simulink subsystem "Channel_FIFO"  (R2024a)
settings: Solver=VariableStepAuto  StartTime=0.0  StopTime=10.0  RelTol=1e-3
model mask{Index=0}
libraries: hdlsllib x2, simulink x1
settings Model: Creator=versal  LastModifiedBy=versal

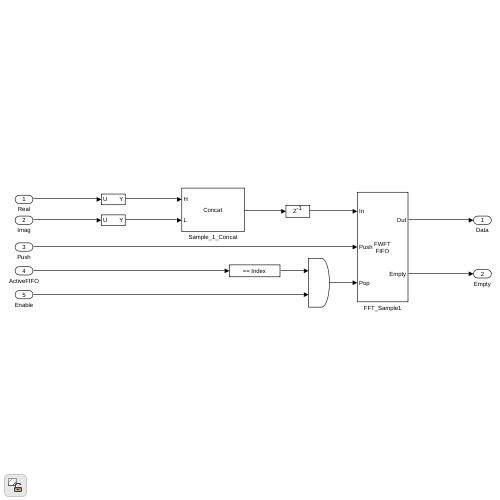
[thumbnail: Simulink's stored preview of the top-level diagram]
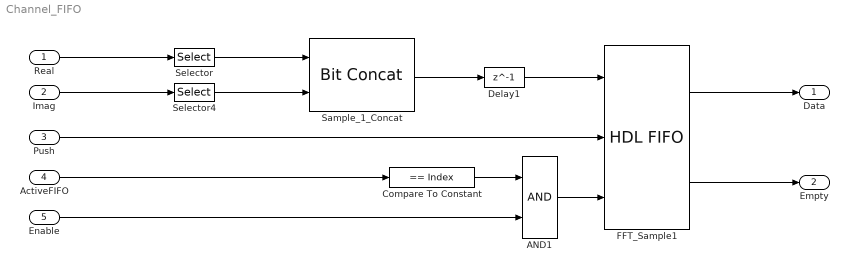
== system Channel_FIFO ==
  Real : Inport
  Imag : Inport  Port=2
  Push : Inport  Port=3
  ActiveFIFO : Inport  Port=4
  Enable : Inport  Port=5
  AND1 : Logic  IconShape=distinctive  AllPortsSameDT=off  OutDataTypeStr=boolean
  Compare To Constant : simulink/Logic and Bit Operations/Compare To Constant  relop===  const=Index  OutDataTypeStr=boolean
  Delay1 : Delay  DelayLength=1
  FFT_Sample1 : hdlsllib/HDL RAMs/HDL FIFO  fifo_size=128  mode=FWFT  ratio=1  push_msg=Warning  pop_msg=Warning  show_empty=on  show_full=off  show_num=off  LabelModeActiveChoice_Mode=FWFT  rst_port=off
  Sample_1_Concat : hdlsllib/Logic and Bit Operations/Bit Concat  numInputs=2
  Selector : Selector  IndexMode=Zero-based  InputPortWidth=16  IndexOptions=Index vector (dialog)  Indices=Index  OutputSizes=1
  Selector4 : Selector  IndexMode=Zero-based  InputPortWidth=16  IndexOptions=Index vector (dialog)  Indices=Index  OutputSizes=1
  Data : Outport
  Empty : Outport  Port=2
  wires:
  Selector/1 -> Sample_1_Concat/1
  Delay1/1 -> FFT_Sample1/1
  Real/1 -> Selector/1
  AND1/1 -> FFT_Sample1/3
  Compare To Constant/1 -> AND1/1
  Selector4/1 -> Sample_1_Concat/2
  ActiveFIFO/1 -> Compare To Constant/1
  Imag/1 -> Selector4/1
  FFT_Sample1/2 -> Empty/1
  Sample_1_Concat/1 -> Delay1/1
  Push/1 -> FFT_Sample1/2
  FFT_Sample1/1 -> Data/1
  Enable/1 -> AND1/2
